simulink library "EnergyLimiter"  (R2022b)
settings: Solver=VariableStepAuto  StartTime=0.0  StopTime=10.0  RelTol=1e-3
values from neighbouring files (symbols this model uses):
  CurrentGainVal = 1.0    (= 1)    [EnergyLimiterConfig.m]    (also in EnergyLimiter_Init.m)
  EnableGainLimiter = 1.0    (= 1)    [EnergyLimiterConfig.m]    (also in EnergyLimiter_Init.m)
  EnergyAdjustmentFactorIndB = 0    [EnergyLimiter_Init.m]
  EnergyMeasurementTimeConstantInSeconds = 0.4    [EnergyLimiterConfig.m]    (also in EnergyLimiter_Init.m)
  frameSize = sys_defs.frameSize_samples    [PhaseDetector_init.m]    (also in PoolDelayCodeGen.m = int32(frameSize); PoolDelaySim.m = int32(frameSize))
  GainChangeStepIndB = 0.5    [EnergyLimiter_Init.m]
  GainDecreaseDurationInSeconds = 0.5    [EnergyLimiterConfig.m]    (also in EnergyLimiter_Init.m)
  GainIncreaseDurationInSeconds = 0.5    [EnergyLimiterConfig.m]    (also in EnergyLimiter_Init.m)
  MaxChannels = 8    [EnergyLimiterConfig.m]    (also in EnergyLimiter_Init.m)
  MaxEnergyLevelIndB = -3    [EnergyLimiter_Init.m]
  MaxGainReductionIndB = 6    [EnergyLimiter_Init.m]
undefined symbols (not defined in the file or in its folder): sample_rate_in_hertz
libraries: EnergyLimiterBtc x1
settings Model: Creator=nikunj.tapodhan  LastModifiedBy=kl13806
settings SolverCC: AlgebraicLoopSolver=TrustRegion
settings DebuggingCC: UnconnectedInputMsg=warning  UnconnectedOutputMsg=warning  UnconnectedLineMsg=warning  SFMachineParentedDataDiag=warning  ArithmeticOperatorsInVariantConditions=warning
settings ModelReferenceCC: EnableRefExpFcnMdlSchedulingChecks=on
settings SFSimCC: CustomCodeUndefinedFunction=UseInterfaceOnly
settings RTWCC: DLArmComputeVersion=19.05

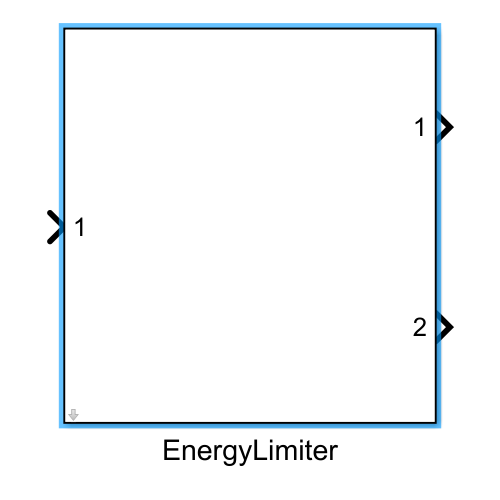
[thumbnail: Simulink's stored preview of the top-level diagram]
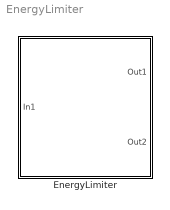
== system EnergyLimiter ==
  EnergyLimiter : Subsystem  mask{EnableGainLimiter=EnableGainLimiter, EnergyMeasurementTimeConstantInSeconds=EnergyMeasurementTimeConstantInSeconds, GainChangeStepIndB=GainChangeStepIndB, MaxEnergyLevelIndB=MaxEnergyLevelIndB, EnergyAdjustmentFactorIndB=EnergyAdjustmentFactorIndB, MaxChannels=MaxChannels, GainIncreaseDurationInSeconds=GainIncreaseDurationInSeconds, GainDecreaseDurationInSeconds=GainDecreaseDurationInSeconds, MaxGainReductionIndB=MaxGainReductionIndB, sample_rate_in_hertz=sample_rate_in_hertz, frameSize=frameSize, CurrentGainVal=CurrentGainVal}
      mask help:
      | This block is used for reducing the gain of an audio signal based upon the crest factor of that signal. Such an algorithm is required for the new generations of amplifiers that have many output channels.
      |
      | Note:Please refer and click on Help tab to get details on configuration parameters
      mask init:
      | blkh = gcbh;
      | % Copy discrete mask parameters into a classdef object
      | InnerLinkConfig = EnergyLimiterConfig;
      | InnerLinkConfig.EnableGainLimiter = EnableGainLimiter;
      | InnerLinkConfig.EnergyMeasurementTimeConstantInSeconds = EnergyMeasurementTimeConstantInSeconds;
      | InnerLinkConfig.GainChangeStepInDb = GainChangeStepIndB;
      | InnerLinkConfig.MaxEnergyLevelInDb = MaxEnergyLevelIndB;
      | InnerLinkConfig.EnergyAdjustmentFactorInDb = EnergyAdjustmentFactorIndB;
      | InnerLinkConfig.MaxChannels = MaxChannels;
      | InnerLinkConfig.GainIncreaseDurationInSeconds = GainIncreaseDurationInSeconds;
      | InnerLinkConfig.GainDecreaseDurationInSeconds = GainDecreaseDurationInSeconds;
      | InnerLinkConfig.MaxGainReductionInDb = MaxGainReductionIndB;
      | 
      | % ----------- BASE WORKSPACE VARIABLES!
      | % Hmm.... the mask does not mention these variables that come from the base
      | % workspace!!! Added them to legacy mask so they will be evaluated from
      | % "wherever" and entered here
      | InnerLinkConfig.Fs = sample_rate_in_hertz;
      | InnerLinkConfig.FrameSize = frameSize;
      | InnerLinkConfig.CurrentGainVal = CurrentGainVal;
      mask Help:
      | Configuration Parameters:
      | 
      |   GainChangeStepIndB
      |                         : Step in dB that gain should be changed by each time signal
      |                           crosses energy threshold. This number should be >= 0.
      | 
      |   GainIncreaseDurationInSeconds
      |                         : Duration that a gain increase should be applied before it
      |                           can be updated. This number should be > 0.
      | 
      |   GainDecreaseDurationInSeconds
      |                         : Duration that a gain decrease should be applied before it
      |                           can be updated. This number should be > 0.
      | 
      |   MaxEnergyLevelIndB
      |                         : Max energy level in dB for each channel above which gain
      |                           energy reduction should kick in. This number should be <= 0
      | 
      |   MaxChannels : Maximum number of channels that may be above energy level
      |                           threshold before gain reduction kicks in.
      |                           This number should be between 0 and numIn (inclusive).
      | 
      |   MaxGainReductionIndB
      |                         : Max gain reduction that should be done.
      |                           This number should be >= 0
      | 
      |   EnergyMeasurementTimeConstantInSeconds
      |                         : Time interval for averaging measured energy (in seconds).
      | 
      |   EnergyAdjustmentFactorIndB
      |                         : A Multiplier factor to adjust EBL threshold based on platform.
      |                           This number should be > 0.
      mask DialogControl Container3 Prompt: Previously undeclared variables

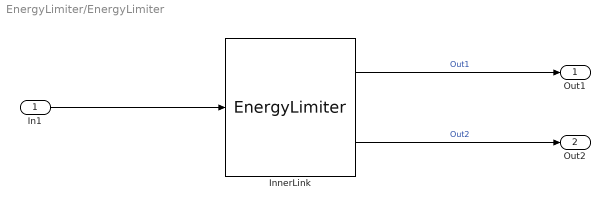
== system EnergyLimiter/EnergyLimiter ==
  In1 : Inport
  InnerLink : EnergyLimiterBtc/EnergyLimiter  Config=InnerLinkConfig  FeatureName=EnergyLimiterSubsystem
      settings: SourceProductName=Bose Blocklib
  Out1 : Outport
  Out2 : Outport  Port=2
  wires:
  InnerLink/1 -> Out1/1  "Out1"
  InnerLink/2 -> Out2/1  "Out2"
  In1/1 -> InnerLink/1
